simulink library "CommercialVehicleLibrary2G"  (R2021a)
settings: Solver=VariableStepAuto  StartTime=0.0  StopTime=10.0  RelTol=1e-3
values from neighbouring files (symbols this model uses):
  brake_input = [0   tmax ... (first row only)    [init_vehicle.m]    (also in run_Circle.m = [0  tmax; run_Coastdown.m = [0  2  tmax; run_DoubleLaneChangeDriver.m = [0   2  tmax; run_MaxAcc.m = [0  2  tmax)
  pose_t0 = [0 0 0 0]    [init_vehicle.m]    (also in run_Circle.m; run_Coastdown.m; run_DoubleLaneChangeDriver.m; run_MaxAcc.m)
  rdfname = 'TNO_FlatRoad.rdf'    [run_Circle.m]    (also in run_Coastdown.m; run_DoubleLaneChangeDriver.m; run_MaxAcc.m; run_Rollover.m)
  rdfname_inner = 'TNO_FlatRoad.rdf'    [run_Circle.m]    (also in run_Coastdown.m; run_DoubleLaneChangeDriver.m; run_MaxAcc.m; run_Rollover.m)
  steer_input = [0  tmax ... (first row only)    [init_vehicle.m]    (also in run_Circle.m = [0  2   10     13       tmax; run_Coastdown.m = [0 tmax; run_DoubleLaneChangeDriver.m = [0 tmax; run_MaxAcc.m = [0 tmax)
  throttle_input = [0         tmax ... (first row only)    [init_vehicle.m]    (also in run_Circle.m; run_Coastdown.m = [0        10         10.0001 tmax; run_DoubleLaneChangeDriver.m = [0        tmax; run_MaxAcc.m = [0        tmax)
  Vx = 0    [init_vehicle.m]    (also in run_Circle.m = Vx_kmh/3.6; run_Coastdown.m = Vx_kmh/3.6; run_DoubleLaneChangeDriver.m = Vx_kmh/3.6; run_MaxAcc.m)
  Vx_input = [0  tmax ... (first row only)    [init_vehicle.m]    (also in run_Circle.m; run_Coastdown.m = [0 tmax; run_DoubleLaneChangeDriver.m = [0 tmax; run_MaxAcc.m = [0 tmax)
undefined symbols (not defined in the file or in its folder): Drive, Floor, Fzstat, Fzstat1, Fzstat3, l, l_load1, l_load2, lbar, mass_load1, mass_load2, psi_semitrailer, rho, rim_Ixx, rim_Iyy, rim_mass, Steer, steer_path, tpfname, X, x_torsion, xcg, xcg1, xcg2, xcg_front, xcg_rear, xdrive1, xload1, xload2, xpos1, xref, xrev1, Xt0, Y, Yt0, Z
libraries: sm_lib x291, $bdroot x157, nesl_utility x143, vrlib x1
(part 8 of 12)

== system CommercialVehicleLibrary2G/Trailers/Trailer - 3 axle  ==
  Mb_trailer : Inport
  Bus Creator : BusCreator  Inputs=6
  Cameras : Subsystem  Commented=on
      settings: PortSchema="{\"entries\":[{\"content\":{\"sides\":[{\"content\":{\"connectorIds\":[]},\"type\":\"ConnectorPlacement.EquallySpacedRectSide\",\"uuid\":\"a276cb58-0a92-429b-8e88-be3307b37bb7\"},{\"content\":{\"connectorIds\":[],\"side\":\"RIGHT\"},\"type\":\"ConnectorPlacement.EquallySpacedRectSide\",\"uuid\":\"8a90bce0-2fe2-4c94-b803-8b8b0449a6a1\"},{\"content\":{\"connectorIds\":[],\"side\":\"TOP\"},\"type\":\"ConnectorPlacement.EquallySpacedRectSide\",\"uuid\":\"98d3107c-5bc7-4afe-b9f8-41acdc56c58c\"},{\"content\":{\"connectorIds\":[\"RConn1\"],\"side\":\"BOTTOM\"},\"type\":\"ConnectorPlacement.EquallySpacedRectSide\",\"uuid\":\"4e4e33e6-8433-45a0-a537-d9ee13bc0975\"}]},\"type\":\"ConnectorPlacement.EquallySpacedConnector\",\"uuid\":\"603d60ad-e553-44b7-87a5-94eb629e36a6\"}],\"packageUris\":[\"http://schema.mathworks.com/mf0/Connector/R2020b\"],\"version\":\"1.0\"}"
  Drawbar joint 1 : $bdroot/Components/Drawbar joint   SystemSampleTime=-1  VariantActivationTime=update diagram  Latency=0  AutoFrameSizeCalculation=off
  To origin : sm_lib/Frames and Transforms/Rigid Transform  TranslationMethod=Cartesian  TranslationStandardOffset=0  TranslationLengthUnit=m  TranslationStandardAxis=+Z  TranslationCartesianOffset=[-xcg2 0 -1.2]  TranslationROffset=0  TranslationROffsetUnits=m  TranslationZOffset=0  TranslationZOffsetUnits=m  TranslationThetaOffset=0  TranslationThetaOffsetUnits=deg  RotationMethod=None  RotationAngleUnits=deg  RotationStandardAxis=+Z  RotationAngle=0.0  RotationArbitraryAxis=[0 0 1]  FollAlignAxisA=+X  BaseAlignAxisA=+Y  FollAlignAxisB=+Y  BaseAlignAxisB=+Z  RotationSequenceAxes=FollowerAxes  RotationSequence=XYX  RotationSequenceAngles=[0 0 0]  RotationSequenceAnglesUnits=deg  RotationMatrix=[1 0 0; 0 1 0; 0 0 1]
  Trailer axle 1 : $bdroot/Assemblies/Trailer axle  xpos=0+xcg2  tpfname='truck3.tpf'  rdfname=rdfname  Vx=Vx  Fzstat=Fzstat
  Trailer axle 2 : $bdroot/Assemblies/Trailer axle  xpos=xpos2  tpfname='truck3.tpf'  rdfname=rdfname  Vx=Vx  Fzstat=Fzstat
  Trailer axle 3 : $bdroot/Assemblies/Trailer axle  xpos=xpos3  tpfname='truck3.tpf'  rdfname=rdfname  Vx=Vx  Fzstat=Fzstat
  Trailer load center : $bdroot/Assemblies/Trailer load center  xload=xcg1  zload=1.3  mass_load=0.5*mass_load  l_load=0.50*l_chassis  w=2.5  rho=rho
  Trailer load center1 : $bdroot/Assemblies/Trailer load center  xload=xcg2  zload=1.3  mass_load=0.5*mass_load  l_load=0.50*l_chassis  w=2.5  rho=rho
  Trailer_front : sm_lib/Body Elements/Brick Solid  GraphicAmbientColor=[0.15 0.15 0.15 1.0]  BasedOnType=Density  BrickDimensions=[l w h]  BrickDimensionUnits=m  CenterOfMass=[0 0 0]  CenterOfMassUnits=m  GraphicDiffuseColor=[0.9 0.9 0.9]  Density=1000  DensityUnits=kg/m^3  DoExposeReferenceFrame=on  GraphicEmissiveColor=[0.0 0.0 0.0 1.0]  ExportEntireGeometry=off  SerializedFrames=<Frames><Frame><Id>Frame1</Id><Value><Name>F1</Name><Origin><Source>ReferenceFrame</Source><FeatureName></FeatureName></Origin><PrimaryAxis><DefinedDirection>+Z</DefinedDirection><Source>ReferenceFrame</Source><SourceDirection>+Z</SourceDirection><FeatureName></FeatureName></PrimaryAxis><SecondaryAxis><DefinedDirection>+X</DefinedDirection><Source>ReferenceFrame</Source><SourceDirection>+X</SourceDirection><FeatureName></FeatureName></SecondaryAxis></Value></Frame></Frames>  MarkerShape=Sphere  MarkerSize=10  GraphicType=FromGeometry  InertiaType=Custom  Mass=chassis_mass  MassUnits=kg  MomentsOfInertia=[chassis_Ixx chassis_Iyy chassis_Izz]  MomentsOfInertiaUnits=kg*m^2  GraphicOpacity=0.8  ProductsOfInertia=[0 0 0]  ProductsOfInertiaUnits=kg*m^2  GraphicShininess=75  GraphicSpecularColor=[0.5 0.5 0.5 1.0]  GraphicVisPropType=SimpleVisualProperties
  Trailer_rear : sm_lib/Body Elements/Brick Solid  GraphicAmbientColor=[0.15 0.15 0.15 1.0]  BasedOnType=Density  BrickDimensions=[l w h]  BrickDimensionUnits=m  CenterOfMass=[0 0 0]  CenterOfMassUnits=m  GraphicDiffuseColor=[0.9 0.9 0.9]  Density=1000  DensityUnits=kg/m^3  DoExposeReferenceFrame=on  GraphicEmissiveColor=[0.0 0.0 0.0 1.0]  ExportEntireGeometry=off  SerializedFrames=<Frames><Frame><Id>Frame1</Id><Value><Name>F1</Name><Origin><Source>ReferenceFrame</Source><FeatureName></FeatureName></Origin><PrimaryAxis><DefinedDirection>+Z</DefinedDirection><Source>ReferenceFrame</Source><SourceDirection>+Z</SourceDirection><FeatureName></FeatureName></PrimaryAxis><SecondaryAxis><DefinedDirection>+X</DefinedDirection><Source>ReferenceFrame</Source><SourceDirection>+X</SourceDirection><FeatureName></FeatureName></SecondaryAxis></Value></Frame></Frames>  MarkerShape=Sphere  MarkerSize=10  GraphicType=FromGeometry  InertiaType=Custom  Mass=chassis_mass  MassUnits=kg  MomentsOfInertia=[chassis_Ixx chassis_Iyy chassis_Izz]  MomentsOfInertiaUnits=kg*m^2  GraphicOpacity=0.8  ProductsOfInertia=[0 0 0]  ProductsOfInertiaUnits=kg*m^2  GraphicShininess=75  GraphicSpecularColor=[0.5 0.5 0.5 1.0]  GraphicVisPropType=SimpleVisualProperties
  Trailer_torsion : $bdroot/Components/Trailer_torsion  SystemSampleTime=-1  VariantActivationTime=update diagram  Latency=0  AutoFrameSizeCalculation=off
      settings: PortSchema="{\"entries\":[{\"content\":{\"sides\":[{\"content\":{\"connectorIds\":[\"LConn1\"]},\"type\":\"ConnectorPlacement.EquallySpacedRectSide\",\"uuid\":\"b43c74bd-af15-4ffb-863b-6a132848d787\"},{\"content\":{\"connectorIds\":[\"RConn1\"],\"side\":\"RIGHT\"},\"type\":\"ConnectorPlacement.EquallySpacedRectSide\",\"uuid\":\"8ef5ae9f-2f99-4b38-816f-c2fb0756fe1b\"},{\"content\":{\"connectorIds\":[\"Out1\"],\"side\":\"TOP\"},\"type\":\"ConnectorPlacement.EquallySpacedRectSide\",\"uuid\":\"649c363b-e78d-45fa-ac8c-bda3eda724e3\"}]},\"type\":\"ConnectorPlacement.EquallySpacedConnector\",\"uuid\":\"06fb9ebd-5177-4420-93bb-82569f181fb4\"}],\"packageUris\":[\"http://schema.mathworks.com/mf0/Connector/R2020b\"],\"version\":\"1.0\"}"
  Pin Coupling : PMIOPort  Tag=PMCPort  Side=Left
  Connection : PMIOPort  Tag=PMCPort  Port=2  Side=Right
  Signals : Outport
  wires:
  [axle2] -> Bus Creator/2  "axle2"
  [axle1] -> Bus Creator/1  "axle1"
  Bus Creator/1 -> Signals/1
  Trailer load center1/1 -> [semitrailerload2]
  Trailer_torsion/1 -> [torsion]
  Mb_trailer/1 -> Trailer axle 1/1, Trailer axle 2/1, Trailer axle 3/1
  Trailer axle 2/1 -> [axle2]
  Trailer load center/1 -> [semitrailerload1]
  Trailer axle 1/1 -> [axle1]
  Trailer axle 3/1 -> [axle3]
  [semitrailerload1] -> Bus Creator/4  "load1"
  [semitrailerload2] -> Bus Creator/5  "load2"
  [torsion] -> Bus Creator/6  "torsion"
  [axle3] -> Bus Creator/3  "axle3"
  connections:
  To origin/LConn1 -- Trailer load center1/LConn1 -- Trailer axle 2/LConn1 -- Trailer axle 3/LConn1 -- Trailer_rear/LConn1
  Cameras/RConn1 -- Trailer_front/LConn1 -- Trailer_torsion/LConn1 -- Trailer load center/LConn1
  Trailer_rear/RConn1 -- Trailer_torsion/RConn1
  To origin/RConn1 -- Connection/RConn1
  Pin Coupling/RConn1 -- Drawbar joint 1/LConn1
  Drawbar joint 1/RConn1 -- Trailer_front/RConn1
  Drawbar joint 1/RConn2 -- Trailer axle 1/LConn1

== system CommercialVehicleLibrary2G/Utilities/Differentiator//filter ==
  pos : Inport
  Gain : Gain  Gain=c  SaturateOnIntegerOverflow=on  OutDataTypeStr=Inherit: Same as input  ParamDataTypeStr=Inherit: Same as input
  Gain2 : Gain  Gain=2*sqrt(c)  SaturateOnIntegerOverflow=on  OutDataTypeStr=Inherit: Same as input  ParamDataTypeStr=Inherit: Same as input
  Integrator2 : Integrator
  Integrator3 : Integrator
  Sum1 : Sum  Inputs=-+|  SaturateOnIntegerOverflow=on
  Sum2 : Sum  Inputs=-+|  SaturateOnIntegerOverflow=on
  actual pos : Outport
  wires:
  Integrator2/1 -> Integrator3/1, Gain2/1
  Integrator3/1 -> Sum2/1, actual pos/1
  Sum1/1 -> Integrator2/1
  Sum2/1 -> Gain/1
  pos/1 -> Sum2/2
  Gain2/1 -> Sum1/1
  Gain/1 -> Sum1/2

== system CommercialVehicleLibrary2G/Utilities/Non-moving road ==
  omega2 : Constant  Value=zeros(18,1)
  road : Outport
  wires:
  omega2/1 -> road/1

== system CommercialVehicleLibrary2G/Utilities/Scaling factors ==
  s_LKX : Constant  Value=LKX
  s_LKY : Constant  Value=LKY
  s_LKYC : Constant  Value=LKYC
  s_LKZC : Constant  Value=LKZC
  s_LMUX : Constant  Value=LMUX
  s_LMUY : Constant  Value=LMUY
  s_LTR : Constant  Value=LTR
  scaling_vector : Mux  Inputs=7
  scaling : Outport
  wires:
  s_LMUX/1 -> scaling_vector/1
  s_LKX/1 -> scaling_vector/2
  s_LMUY/1 -> scaling_vector/3
  s_LKY/1 -> scaling_vector/4
  s_LKYC/1 -> scaling_vector/5
  s_LTR/1 -> scaling_vector/6
  s_LKZC/1 -> scaling_vector/7
  scaling_vector/1 -> scaling/1

== system CommercialVehicleLibrary2G/Utilities/To_workspace_dolly ==
  note: Axle 1
  note: Axle 2
  note: Tyres & Omega
  In1 : Inport
  Bus Selector10 : BusSelector  OutputSignals=axle1.Axle_roll  OutputAsBus=on
  Bus Selector12 : BusSelector  OutputSignals=axle2.Axle_acc  OutputAsBus=on
  Bus Selector2 : BusSelector  OutputSignals=axle2.Axle_pos  OutputAsBus=on
  Bus Selector3 : BusSelector  OutputSignals=axle2.Axle_roll  OutputAsBus=on
  Bus Selector5 : BusSelector  OutputSignals=axle1.Axle_pos  OutputAsBus=on
  Bus Selector6 : BusSelector  OutputSignals=axle1.Axle_acc  OutputAsBus=on
  Subsystem : Subsystem
  Subsystem1 : Subsystem
  Subsystem2 : Subsystem
  Subsystem3 : Subsystem
  To Workspace10 : ToWorkspace  VariableName=p_trailer1_axle2_acc  SampleTime=-1
  To Workspace23 : ToWorkspace  VariableName=p_trailer1_axle1_roll  SampleTime=-1
  To Workspace30 : ToWorkspace  VariableName=p_trailer1_Fx  SampleTime=-1
  To Workspace31 : ToWorkspace  VariableName=p_trailer1_Fy  SampleTime=-1
  To Workspace4 : ToWorkspace  VariableName=p_trailer1_axle2_roll  SampleTime=-1
  To Workspace5 : ToWorkspace  VariableName=p_trailer1_axle1_pos  SampleTime=-1
  To Workspace6 : ToWorkspace  VariableName=p_trailer1_axle1_acc  SampleTime=-1
  To Workspace7 : ToWorkspace  VariableName=p_trailer1_omega  SampleTime=-1
  To Workspace8 : ToWorkspace  VariableName=p_trailer1_axle2_pos  SampleTime=-1
  To Workspace9 : ToWorkspace  VariableName=p_trailer1_Fz  SampleTime=-1
  wires:
  Bus Selector10/1 -> To Workspace23/1
  In1/1 -> Bus Selector3/1, Bus Selector2/1, Bus Selector5/1, Bus Selector12/1, Bus Selector10/1, Subsystem3/1(In1), Subsystem2/1(In1), Subsystem1/1(In1), Subsystem/1(In1), Bus Selector6/1
  Bus Selector12/1 -> To Workspace10/1
  Bus Selector6/1 -> To Workspace6/1
  Bus Selector5/1 -> To Workspace5/1
  Subsystem3/1(Out1) -> To Workspace7/1
  Subsystem2/1(Out1) -> To Workspace9/1
  Subsystem1/1(Out1) -> To Workspace31/1
  Subsystem/1(Out1) -> To Workspace30/1
  Bus Selector3/1 -> To Workspace4/1
  Bus Selector2/1 -> To Workspace8/1

== system CommercialVehicleLibrary2G/Utilities/To_workspace_drawbar_trailer_2axle ==
  note: Axle 1
  note: Axle 2
  note: Chassis & Load
  note: Tyres & Omega
  In1 : Inport
  Bus Selector10 : BusSelector  OutputSignals=axle1.Axle_roll  OutputAsBus=on
  Bus Selector11 : BusSelector  OutputSignals=trailerload.acc_center  OutputAsBus=on
  Bus Selector12 : BusSelector  OutputSignals=axle2.Axle_acc  OutputAsBus=on
  Bus Selector2 : BusSelector  OutputSignals=axle2.Axle_pos  OutputAsBus=on
  Bus Selector22 : BusSelector  OutputSignals=trailerload.pos  OutputAsBus=on
  Bus Selector3 : BusSelector  OutputSignals=axle2.Axle_roll  OutputAsBus=on
  Bus Selector5 : BusSelector  OutputSignals=axle1.Axle_pos  OutputAsBus=on
  Bus Selector6 : BusSelector  OutputSignals=axle1.Axle_acc  OutputAsBus=on
  Bus Selector7 : BusSelector  OutputSignals=trailerload.acc_corner  OutputAsBus=on
  Subsystem : Subsystem
  Subsystem1 : Subsystem
  Subsystem2 : Subsystem
  Subsystem3 : Subsystem
  To Workspace1 : ToWorkspace  VariableName=p_trailer1_load_pos  SampleTime=-1
  To Workspace10 : ToWorkspace  VariableName=p_trailer1_axle2_acc  SampleTime=-1
  To Workspace2 : ToWorkspace  VariableName=p_trailer1_load_acc_center  SampleTime=-1
  To Workspace23 : ToWorkspace  VariableName=p_trailer1_axle1_roll  SampleTime=-1
  To Workspace3 : ToWorkspace  VariableName=p_trailer1_load_acc_corner  SampleTime=-1
  To Workspace30 : ToWorkspace  VariableName=p_trailer1_Fx  SampleTime=-1
  To Workspace31 : ToWorkspace  VariableName=p_trailer1_Fy  SampleTime=-1
  To Workspace4 : ToWorkspace  VariableName=p_trailer1_axle2_roll  SampleTime=-1
  To Workspace5 : ToWorkspace  VariableName=p_trailer1_axle1_pos  SampleTime=-1
  To Workspace6 : ToWorkspace  VariableName=p_trailer1_axle1_acc  SampleTime=-1
  To Workspace7 : ToWorkspace  VariableName=p_trailer1_omega  SampleTime=-1
  To Workspace8 : ToWorkspace  VariableName=p_trailer1_axle2_pos  SampleTime=-1
  To Workspace9 : ToWorkspace  VariableName=p_trailer1_Fz  SampleTime=-1
  wires:
  Bus Selector7/1 -> To Workspace3/1
  Bus Selector10/1 -> To Workspace23/1
  Bus Selector22/1 -> To Workspace1/1
  In1/1 -> Bus Selector3/1, Bus Selector2/1, Bus Selector5/1, Bus Selector12/1, Bus Selector10/1, Subsystem3/1(In1), Bus Selector7/1, Subsystem2/1(In1), Subsystem1/1(In1), Bus Selector22/1, Subsystem/1(In1), Bus Selector11/1, Bus Selector6/1
  Bus Selector12/1 -> To Workspace10/1
  Bus Selector6/1 -> To Workspace6/1
  Bus Selector5/1 -> To Workspace5/1
  Subsystem3/1(Out1) -> To Workspace7/1
  Subsystem2/1(Out1) -> To Workspace9/1
  Subsystem1/1(Out1) -> To Workspace31/1
  Subsystem/1(Out1) -> To Workspace30/1
  Bus Selector3/1 -> To Workspace4/1
  Bus Selector2/1 -> To Workspace8/1
  Bus Selector11/1 -> To Workspace2/1

== system CommercialVehicleLibrary2G/Utilities/To_workspace_drawbar_trailer_3axle ==
  note: Axle 1
  note: Axle 2
  note: Chassis & Load
  note: Tyres & Omega
  note: Axle 3
  In1 : Inport
  Bus Selector1 : BusSelector  OutputSignals=axle3.Axle_roll  OutputAsBus=on
  Bus Selector10 : BusSelector  OutputSignals=axle1.Axle_roll  OutputAsBus=on
  Bus Selector11 : BusSelector  OutputSignals=trailerload.acc_center  OutputAsBus=on
  Bus Selector12 : BusSelector  OutputSignals=axle2.Axle_acc  OutputAsBus=on
  Bus Selector2 : BusSelector  OutputSignals=axle2.Axle_pos  OutputAsBus=on
  Bus Selector22 : BusSelector  OutputSignals=trailerload.pos  OutputAsBus=on
  Bus Selector3 : BusSelector  OutputSignals=axle2.Axle_roll  OutputAsBus=on
  Bus Selector4 : BusSelector  OutputSignals=axle3.Axle_pos  OutputAsBus=on
  Bus Selector5 : BusSelector  OutputSignals=axle1.Axle_pos  OutputAsBus=on
  Bus Selector6 : BusSelector  OutputSignals=axle1.Axle_acc  OutputAsBus=on
  Bus Selector7 : BusSelector  OutputSignals=trailerload.acc_corner  OutputAsBus=on
  Bus Selector8 : BusSelector  OutputSignals=axle3.Axle_acc  OutputAsBus=on
  Subsystem : Subsystem
  Subsystem1 : Subsystem
  Subsystem2 : Subsystem
  Subsystem3 : Subsystem
  To Workspace1 : ToWorkspace  VariableName=p_trailer1_load_pos  SampleTime=-1
  To Workspace10 : ToWorkspace  VariableName=p_trailer1_axle2_acc  SampleTime=-1
  To Workspace11 : ToWorkspace  VariableName=p_trailer1_axle3_pos  SampleTime=-1
  To Workspace12 : ToWorkspace  VariableName=p_trailer1_axle3_acc  SampleTime=-1
  To Workspace13 : ToWorkspace  VariableName=p_trailer1_load_acc_corner  SampleTime=-1
  To Workspace2 : ToWorkspace  VariableName=p_trailer1_load_acc_center  SampleTime=-1
  To Workspace23 : ToWorkspace  VariableName=p_trailer1_axle1_roll  SampleTime=-1
  To Workspace3 : ToWorkspace  VariableName=p_trailer1_axle3_roll  SampleTime=-1
  To Workspace30 : ToWorkspace  VariableName=p_trailer1_Fx  SampleTime=-1
  To Workspace31 : ToWorkspace  VariableName=p_trailer1_Fy  SampleTime=-1
  To Workspace4 : ToWorkspace  VariableName=p_trailer1_axle2_roll  SampleTime=-1
  To Workspace5 : ToWorkspace  VariableName=p_trailer1_axle1_pos  SampleTime=-1
  To Workspace6 : ToWorkspace  VariableName=p_trailer1_axle1_acc  SampleTime=-1
  To Workspace7 : ToWorkspace  VariableName=p_trailer1_omega  SampleTime=-1
  To Workspace8 : ToWorkspace  VariableName=p_trailer1_axle2_pos  SampleTime=-1
  To Workspace9 : ToWorkspace  VariableName=p_trailer1_Fz  SampleTime=-1
  wires:
  Bus Selector7/1 -> To Workspace13/1
  Bus Selector10/1 -> To Workspace23/1
  Bus Selector22/1 -> To Workspace1/1
  In1/1 -> Bus Selector3/1, Bus Selector2/1, Bus Selector5/1, Bus Selector12/1, Bus Selector10/1, Bus Selector8/1, Bus Selector4/1, Bus Selector1/1, Subsystem3/1(In1), Bus Selector7/1, Subsystem2/1(In1), Subsystem1/1(In1), Bus Selector22/1, Subsystem/1(In1), Bus Selector11/1, Bus Selector6/1
  Bus Selector12/1 -> To Workspace10/1
  Bus Selector6/1 -> To Workspace6/1
  Bus Selector5/1 -> To Workspace5/1
  Subsystem3/1(Out1) -> To Workspace7/1
  Subsystem2/1(Out1) -> To Workspace9/1
  Subsystem1/1(Out1) -> To Workspace31/1
  Subsystem/1(Out1) -> To Workspace30/1
  Bus Selector3/1 -> To Workspace4/1
  Bus Selector2/1 -> To Workspace8/1
  Bus Selector11/1 -> To Workspace2/1
  Bus Selector4/1 -> To Workspace11/1
  Bus Selector8/1 -> To Workspace12/1
  Bus Selector1/1 -> To Workspace3/1

== system CommercialVehicleLibrary2G/Utilities/To_workspace_semitrailer ==
  note: Axle 1
  note: Axle 2
  note: Axle 3
  note: Tyres & Omega
  In1 : Inport
  Bus Selector1 : BusSelector  OutputSignals=axle1.Axle_roll  OutputAsBus=on
  Bus Selector11 : BusSelector  OutputSignals=axle3.Axle_acc  OutputAsBus=on
  Bus Selector2 : BusSelector  OutputSignals=axle2.Axle_pos  OutputAsBus=on
  Bus Selector22 : BusSelector  OutputSignals=axle3.Axle_pos  OutputAsBus=on
  Bus Selector3 : BusSelector  OutputSignals=axle2.Axle_acc  OutputAsBus=on
  Bus Selector4 : BusSelector  OutputSignals=axle2.Axle_roll  OutputAsBus=on
  Bus Selector5 : BusSelector  OutputSignals=axle1.Axle_pos  OutputAsBus=on
  Bus Selector6 : BusSelector  OutputSignals=axle1.Axle_acc  OutputAsBus=on
  Bus Selector7 : BusSelector  OutputSignals=axle3.Axle_roll  OutputAsBus=on
  Subsystem : Subsystem
  Subsystem1 : Subsystem
  Subsystem2 : Subsystem
  Subsystem3 : Subsystem
  To Workspace1 : ToWorkspace  VariableName=p_semitraileraxle3_pos  SampleTime=-1
  To Workspace10 : ToWorkspace  VariableName=p_semitraileraxle2_pos  SampleTime=-1
  To Workspace11 : ToWorkspace  VariableName=p_semitraileraxle2_acc  SampleTime=-1
  To Workspace2 : ToWorkspace  VariableName=p_semitraileraxle3_acc  SampleTime=-1
  To Workspace3 : ToWorkspace  VariableName=p_semitraileraxle3_roll  SampleTime=-1
  To Workspace30 : ToWorkspace  VariableName=p_semitrailer_Fx  SampleTime=-1
  To Workspace31 : ToWorkspace  VariableName=p_semitrailer_Fy  SampleTime=-1
  To Workspace4 : ToWorkspace  VariableName=p_semitraileraxle1_roll  SampleTime=-1
  To Workspace5 : ToWorkspace  VariableName=p_semitraileraxle1_pos  SampleTime=-1
  To Workspace6 : ToWorkspace  VariableName=p_semitraileraxle1_acc  SampleTime=-1
  To Workspace7 : ToWorkspace  VariableName=p_semitrailer_omega  SampleTime=-1
  To Workspace8 : ToWorkspace  VariableName=p_semitraileraxle2_roll  SampleTime=-1
  To Workspace9 : ToWorkspace  VariableName=p_semitrailer_Fz  SampleTime=-1
  wires:
  Bus Selector22/1 -> To Workspace1/1
  Bus Selector6/1 -> To Workspace6/1
  Bus Selector5/1 -> To Workspace5/1
  Subsystem3/1(Out1) -> To Workspace7/1
  Subsystem2/1(Out1) -> To Workspace9/1
  Subsystem1/1(Out1) -> To Workspace31/1
  Subsystem/1(Out1) -> To Workspace30/1
  Bus Selector3/1 -> To Workspace11/1
  Bus Selector2/1 -> To Workspace10/1
  Bus Selector11/1 -> To Workspace2/1
  Bus Selector1/1 -> To Workspace4/1
  Bus Selector4/1 -> To Workspace8/1
  In1/1 -> Bus Selector3/1, Bus Selector2/1, Bus Selector5/1, Bus Selector7/1, Subsystem3/1(In1), Subsystem2/1(In1), Subsystem1/1(In1), Bus Selector22/1, Subsystem/1(In1), Bus Selector11/1, Bus Selector4/1, Bus Selector1/1, Bus Selector6/1
  Bus Selector7/1 -> To Workspace3/1

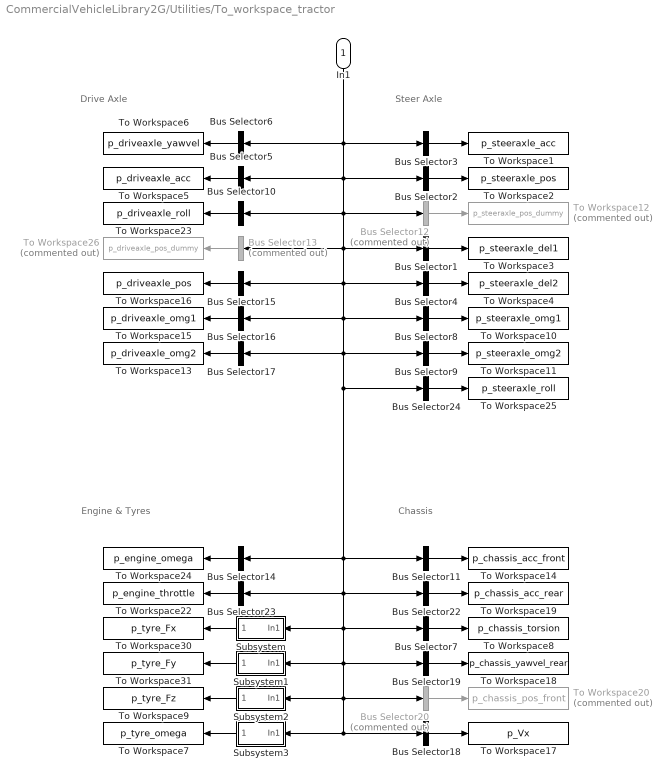
== system CommercialVehicleLibrary2G/Utilities/To_workspace_tractor ==
  note: Drive Axle
  note: Steer Axle
  note: Chassis
  note: Engine & Tyres
  In1 : Inport
  Bus Selector1 : BusSelector  OutputSignals=steeraxle.Delta 1_L  OutputAsBus=on
  Bus Selector10 : BusSelector  OutputSignals=driveaxle.roll  OutputAsBus=on
  Bus Selector11 : BusSelector  OutputSignals=chassis.front_acc  OutputAsBus=on
  Bus Selector12 : BusSelector  Commented=on  OutputSignals=steeraxle.Dummyaxle_pos  OutputAsBus=on
  Bus Selector13 : BusSelector  Commented=on  OutputSignals=driveaxle.G2_Driveaxle_pos_dummy  OutputAsBus=on
  Bus Selector14 : BusSelector  OutputSignals=driveline.omega  OutputAsBus=on
  Bus Selector15 : BusSelector  OutputSignals=driveaxle.pos  OutputAsBus=on
  Bus Selector16 : BusSelector  OutputSignals=driveaxle.Omega1  OutputAsBus=on
  Bus Selector17 : BusSelector  OutputSignals=driveaxle.Omega2  OutputAsBus=on
  Bus Selector18 : BusSelector  OutputSignals=chassis.Vx  OutputAsBus=on
  Bus Selector19 : BusSelector  OutputSignals=chassis.yawvel  OutputAsBus=on
  Bus Selector2 : BusSelector  OutputSignals=steeraxle.pos  OutputAsBus=on
  Bus Selector20 : BusSelector  Commented=on  OutputSignals=chassis.pos_chassis frt  OutputAsBus=on
  Bus Selector22 : BusSelector  OutputSignals=chassis.centre_acc  OutputAsBus=on
  Bus Selector23 : BusSelector  OutputSignals=driveline.throttle  OutputAsBus=on
  Bus Selector24 : BusSelector  OutputSignals=steeraxle.roll  OutputAsBus=on
  Bus Selector3 : BusSelector  OutputSignals=steeraxle.acc  OutputAsBus=on
  Bus Selector4 : BusSelector  OutputSignals=steeraxle.Delta 2_R  OutputAsBus=on
  Bus Selector5 : BusSelector  OutputSignals=driveaxle.acc  OutputAsBus=on
  Bus Selector6 : BusSelector  OutputSignals=chassis.yawvel  OutputAsBus=on
  Bus Selector7 : BusSelector  OutputSignals=chassis.torsion  OutputAsBus=on
  Bus Selector8 : BusSelector  OutputSignals=steeraxle.Omega1  OutputAsBus=on
  Bus Selector9 : BusSelector  OutputSignals=steeraxle.Omega2  OutputAsBus=on
  Subsystem : Subsystem
  Subsystem1 : Subsystem
  Subsystem2 : Subsystem
  Subsystem3 : Subsystem
  To Workspace1 : ToWorkspace  VariableName=p_steeraxle_acc  SampleTime=-1
  To Workspace10 : ToWorkspace  VariableName=p_steeraxle_omg1  SampleTime=-1
  To Workspace11 : ToWorkspace  VariableName=p_steeraxle_omg2  SampleTime=-1
  To Workspace12 : ToWorkspace  Commented=on  VariableName=p_steeraxle_pos_dummy  SampleTime=-1
  To Workspace13 : ToWorkspace  VariableName=p_driveaxle_omg2  SampleTime=-1
  To Workspace14 : ToWorkspace  VariableName=p_chassis_acc_front  SampleTime=-1
  To Workspace15 : ToWorkspace  VariableName=p_driveaxle_omg1  SampleTime=-1
  To Workspace16 : ToWorkspace  VariableName=p_driveaxle_pos  SampleTime=-1
  To Workspace17 : ToWorkspace  VariableName=p_Vx  SampleTime=-1
  To Workspace18 : ToWorkspace  VariableName=p_chassis_yawvel_rear  SampleTime=-1
  To Workspace19 : ToWorkspace  VariableName=p_chassis_acc_rear  SampleTime=-1
  To Workspace2 : ToWorkspace  VariableName=p_steeraxle_pos  SampleTime=-1
  To Workspace20 : ToWorkspace  Commented=on  VariableName=p_chassis_pos_front  SampleTime=-1
  To Workspace22 : ToWorkspace  VariableName=p_engine_throttle  SampleTime=-1
  To Workspace23 : ToWorkspace  VariableName=p_driveaxle_roll  SampleTime=-1
  To Workspace24 : ToWorkspace  VariableName=p_engine_omega  SampleTime=-1
  To Workspace25 : ToWorkspace  VariableName=p_steeraxle_roll  SampleTime=-1
  To Workspace26 : ToWorkspace  Commented=on  VariableName=p_driveaxle_pos_dummy  SampleTime=-1
  To Workspace3 : ToWorkspace  VariableName=p_steeraxle_del1  SampleTime=-1
  To Workspace30 : ToWorkspace  VariableName=p_tyre_Fx  SampleTime=-1
  To Workspace31 : ToWorkspace  VariableName=p_tyre_Fy  SampleTime=-1
  To Workspace4 : ToWorkspace  VariableName=p_steeraxle_del2  SampleTime=-1
  To Workspace5 : ToWorkspace  VariableName=p_driveaxle_acc  SampleTime=-1
  To Workspace6 : ToWorkspace  VariableName=p_driveaxle_yawvel  SampleTime=-1
  To Workspace7 : ToWorkspace  VariableName=p_tyre_omega  SampleTime=-1
  To Workspace8 : ToWorkspace  VariableName=p_chassis_torsion  SampleTime=-1
  To Workspace9 : ToWorkspace  VariableName=p_tyre_Fz  SampleTime=-1
  wires:
  Bus Selector13/1 -> To Workspace26/1
  Bus Selector24/1 -> To Workspace25/1
  Bus Selector10/1 -> To Workspace23/1
  Bus Selector23/1 -> To Workspace22/1
  Bus Selector20/1 -> To Workspace20/1
  In1/1 -> Bus Selector3/1, Bus Selector2/1, Bus Selector5/1, Bus Selector12/1, Bus Selector10/1, Bus Selector1/1, Bus Selector13/1, Bus Selector4/1, Bus Selector15/1, Bus Selector8/1, Bus Selector16/1, Bus Selector9/1, Bus Selector17/1, Bus Selector11/1, Bus Selector14/1, Bus Selector22/1, Bus Selector7/1, Subsystem/1(In1), Bus Selector19/1, Subsystem1/1(In1), Bus Selector20/1, Subsystem2/1(In1), Subsystem3/1(In1), Bus Selector18/1, Bus Selector23/1, Bus Selector24/1, Bus Selector6/1
  Bus Selector22/1 -> To Workspace19/1
  Bus Selector19/1 -> To Workspace18/1
  Bus Selector15/1 -> To Workspace16/1
  Bus Selector17/1 -> To Workspace13/1
  Bus Selector16/1 -> To Workspace15/1
  Bus Selector12/1 -> To Workspace12/1
  Bus Selector9/1 -> To Workspace11/1
  Bus Selector8/1 -> To Workspace10/1
  Bus Selector6/1 -> To Workspace6/1
  Bus Selector5/1 -> To Workspace5/1
  Bus Selector4/1 -> To Workspace4/1
  Bus Selector1/1 -> To Workspace3/1
  Subsystem3/1(Out1) -> To Workspace7/1
  Subsystem2/1(Out1) -> To Workspace9/1
  Subsystem1/1(Out1) -> To Workspace31/1
  Subsystem/1(Out1) -> To Workspace30/1
  Bus Selector3/1 -> To Workspace1/1
  Bus Selector2/1 -> To Workspace2/1
  Bus Selector7/1 -> To Workspace8/1
  Bus Selector18/1 -> To Workspace17/1
  Bus Selector11/1 -> To Workspace14/1
  Bus Selector14/1 -> To Workspace24/1

== system CommercialVehicleLibrary2G/Utilities/To_workspace_trailer_2axle ==
  note: Axle 1
  note: Axle 2
  note: Chassis & Load
  note: Tyres & Omega
  In1 : Inport
  Bus Selector1 : BusSelector  OutputSignals=load2.acc_center  OutputAsBus=on
  Bus Selector10 : BusSelector  OutputSignals=axle1.Axle_roll  OutputAsBus=on
  Bus Selector11 : BusSelector  OutputSignals=load1.acc_center  OutputAsBus=on
  Bus Selector12 : BusSelector  OutputSignals=axle2.Axle_acc  OutputAsBus=on
  Bus Selector2 : BusSelector  OutputSignals=axle2.Axle_pos  OutputAsBus=on
  Bus Selector22 : BusSelector  OutputSignals=load1.pos  OutputAsBus=on
  Bus Selector3 : BusSelector  OutputSignals=axle2.Axle_roll  OutputAsBus=on
  Bus Selector4 : BusSelector  OutputSignals=load2.pos  OutputAsBus=on
  Bus Selector5 : BusSelector  OutputSignals=axle1.Axle_pos  OutputAsBus=on
  Bus Selector6 : BusSelector  OutputSignals=axle1.Axle_acc  OutputAsBus=on
  Bus Selector7 : BusSelector  OutputSignals=torsion  OutputAsBus=on
  Bus Selector8 : BusSelector  OutputSignals=load1.acc_corner  OutputAsBus=on
  Bus Selector9 : BusSelector  OutputSignals=load2.acc_corner  OutputAsBus=on
  Subsystem : Subsystem
  Subsystem1 : Subsystem
  Subsystem2 : Subsystem
  Subsystem3 : Subsystem
  To Workspace1 : ToWorkspace  VariableName=p_trailer1_load1_pos  SampleTime=-1
  To Workspace10 : ToWorkspace  VariableName=p_trailer1_axle2_acc  SampleTime=-1
  To Workspace11 : ToWorkspace  VariableName=p_trailer1_load2_pos  SampleTime=-1
  To Workspace12 : ToWorkspace  VariableName=p_trailer1_load2_acc_center  SampleTime=-1
  To Workspace13 : ToWorkspace  VariableName=p_trailer1_load1_acc_corner  SampleTime=-1
  To Workspace14 : ToWorkspace  VariableName=p_trailer1_load2_acc_corner  SampleTime=-1
  To Workspace2 : ToWorkspace  VariableName=p_trailer1_load1_acc_center  SampleTime=-1
  To Workspace23 : ToWorkspace  VariableName=p_trailer1_axle1_roll  SampleTime=-1
  To Workspace3 : ToWorkspace  VariableName=p_trailer1_torsion  SampleTime=-1
  To Workspace30 : ToWorkspace  VariableName=p_trailer1_Fx  SampleTime=-1
  To Workspace31 : ToWorkspace  VariableName=p_trailer1_Fy  SampleTime=-1
  To Workspace4 : ToWorkspace  VariableName=p_trailer1_axle2_roll  SampleTime=-1
  To Workspace5 : ToWorkspace  VariableName=p_trailer1_axle1_pos  SampleTime=-1
  To Workspace6 : ToWorkspace  VariableName=p_trailer1_axle1_acc  SampleTime=-1
  To Workspace7 : ToWorkspace  VariableName=p_trailer1_omega  SampleTime=-1
  To Workspace8 : ToWorkspace  VariableName=p_trailer1_axle2_pos  SampleTime=-1
  To Workspace9 : ToWorkspace  VariableName=p_trailer1_Fz  SampleTime=-1
  wires:
  Bus Selector9/1 -> To Workspace14/1
  Bus Selector8/1 -> To Workspace13/1
  Bus Selector10/1 -> To Workspace23/1
  Bus Selector22/1 -> To Workspace1/1
  Bus Selector12/1 -> To Workspace10/1
  Bus Selector6/1 -> To Workspace6/1
  Bus Selector5/1 -> To Workspace5/1
  Subsystem3/1(Out1) -> To Workspace7/1
  Subsystem2/1(Out1) -> To Workspace9/1
  Subsystem1/1(Out1) -> To Workspace31/1
  Subsystem/1(Out1) -> To Workspace30/1
  Bus Selector3/1 -> To Workspace4/1
  Bus Selector2/1 -> To Workspace8/1
  Bus Selector11/1 -> To Workspace2/1
  Bus Selector7/1 -> To Workspace3/1
  Bus Selector1/1 -> To Workspace12/1
  In1/1 -> Bus Selector3/1, Bus Selector2/1, Bus Selector5/1, Bus Selector12/1, Bus Selector10/1, Subsystem1/1(In1), Subsystem2/1(In1), Subsystem3/1(In1), Bus Selector4/1, Bus Selector7/1, Bus Selector9/1, Bus Selector1/1, Bus Selector22/1, Bus Selector8/1, Subsystem/1(In1), Bus Selector11/1, Bus Selector6/1
  Bus Selector4/1 -> To Workspace11/1

== system CommercialVehicleLibrary2G/Utilities/To_workspace_trailer_3axle ==
  note: Axle 1
  note: Axle 2
  note: Chassis & Load
  note: Tyres & Omega
  note: Axle 3
  In1 : Inport
  Bus Selector1 : BusSelector  OutputSignals=load2.acc_center  OutputAsBus=on
  Bus Selector10 : BusSelector  OutputSignals=axle1.Axle_roll  OutputAsBus=on
  Bus Selector11 : BusSelector  OutputSignals=load1.acc_center  OutputAsBus=on
  Bus Selector12 : BusSelector  OutputSignals=axle2.Axle_acc  OutputAsBus=on
  Bus Selector13 : BusSelector  OutputSignals=axle3.Axle_acc  OutputAsBus=on
  Bus Selector14 : BusSelector  OutputSignals=load1.acc_corner  OutputAsBus=on
  Bus Selector15 : BusSelector  OutputSignals=load2.acc_corner  OutputAsBus=on
  Bus Selector2 : BusSelector  OutputSignals=axle2.Axle_pos  OutputAsBus=on
  Bus Selector22 : BusSelector  OutputSignals=load1.pos  OutputAsBus=on
  Bus Selector3 : BusSelector  OutputSignals=axle2.Axle_roll  OutputAsBus=on
  Bus Selector4 : BusSelector  OutputSignals=load2.pos  OutputAsBus=on
  Bus Selector5 : BusSelector  OutputSignals=axle1.Axle_pos  OutputAsBus=on
  Bus Selector6 : BusSelector  OutputSignals=axle1.Axle_acc  OutputAsBus=on
  Bus Selector7 : BusSelector  OutputSignals=torsion  OutputAsBus=on
  Bus Selector8 : BusSelector  OutputSignals=axle3.Axle_roll  OutputAsBus=on
  Bus Selector9 : BusSelector  OutputSignals=axle3.Axle_pos  OutputAsBus=on
  Subsystem : Subsystem
  Subsystem1 : Subsystem
  Subsystem2 : Subsystem
  Subsystem3 : Subsystem
  To Workspace1 : ToWorkspace  VariableName=p_trailer1_load1_pos  SampleTime=-1
  To Workspace10 : ToWorkspace  VariableName=p_trailer1_axle2_acc  SampleTime=-1
  To Workspace11 : ToWorkspace  VariableName=p_trailer1_load2_pos  SampleTime=-1
  To Workspace12 : ToWorkspace  VariableName=p_trailer1_load2_acc_center  SampleTime=-1
  To Workspace13 : ToWorkspace  VariableName=p_trailer1_axle3_roll  SampleTime=-1
  To Workspace14 : ToWorkspace  VariableName=p_trailer1_axle3_pos  SampleTime=-1
  To Workspace15 : ToWorkspace  VariableName=p_trailer1_axle3_acc  SampleTime=-1
  To Workspace16 : ToWorkspace  VariableName=p_trailer1_load1_acc_corner  SampleTime=-1
  To Workspace17 : ToWorkspace  VariableName=p_trailer1_load2_acc_corner  SampleTime=-1
  To Workspace2 : ToWorkspace  VariableName=p_trailer1_load1_acc_center  SampleTime=-1
  To Workspace23 : ToWorkspace  VariableName=p_trailer1_axle1_roll  SampleTime=-1
  To Workspace3 : ToWorkspace  VariableName=p_trailer1_torsion  SampleTime=-1
  To Workspace30 : ToWorkspace  VariableName=p_trailer1_Fx  SampleTime=-1
  To Workspace31 : ToWorkspace  VariableName=p_trailer1_Fy  SampleTime=-1
  To Workspace4 : ToWorkspace  VariableName=p_trailer1_axle2_roll  SampleTime=-1
  To Workspace5 : ToWorkspace  VariableName=p_trailer1_axle1_pos  SampleTime=-1
  To Workspace6 : ToWorkspace  VariableName=p_trailer1_axle1_acc  SampleTime=-1
  To Workspace7 : ToWorkspace  VariableName=p_trailer1_omega  SampleTime=-1
  To Workspace8 : ToWorkspace  VariableName=p_trailer1_axle2_pos  SampleTime=-1
  To Workspace9 : ToWorkspace  VariableName=p_trailer1_Fz  SampleTime=-1
  wires:
  Bus Selector15/1 -> To Workspace17/1
  Bus Selector14/1 -> To Workspace16/1
  Bus Selector10/1 -> To Workspace23/1
  Bus Selector22/1 -> To Workspace1/1
  Bus Selector12/1 -> To Workspace10/1
  Bus Selector6/1 -> To Workspace6/1
  Bus Selector5/1 -> To Workspace5/1
  Subsystem3/1(Out1) -> To Workspace7/1
  Subsystem2/1(Out1) -> To Workspace9/1
  Subsystem1/1(Out1) -> To Workspace31/1
  Subsystem/1(Out1) -> To Workspace30/1
  Bus Selector3/1 -> To Workspace4/1
  Bus Selector2/1 -> To Workspace8/1
  Bus Selector11/1 -> To Workspace2/1
  Bus Selector7/1 -> To Workspace3/1
  Bus Selector1/1 -> To Workspace12/1
  In1/1 -> Bus Selector3/1, Bus Selector2/1, Bus Selector5/1, Bus Selector12/1, Bus Selector10/1, Bus Selector13/1, Bus Selector11/1, Bus Selector9/1, Bus Selector8/1, Bus Selector22/1, Bus Selector1/1, Bus Selector15/1, Bus Selector4/1, Subsystem2/1(In1), Subsystem3/1(In1), Bus Selector7/1, Subsystem1/1(In1), Subsystem/1(In1), Bus Selector14/1, Bus Selector6/1
  Bus Selector4/1 -> To Workspace11/1
  Bus Selector9/1 -> To Workspace14/1
  Bus Selector13/1 -> To Workspace15/1
  Bus Selector8/1 -> To Workspace13/1

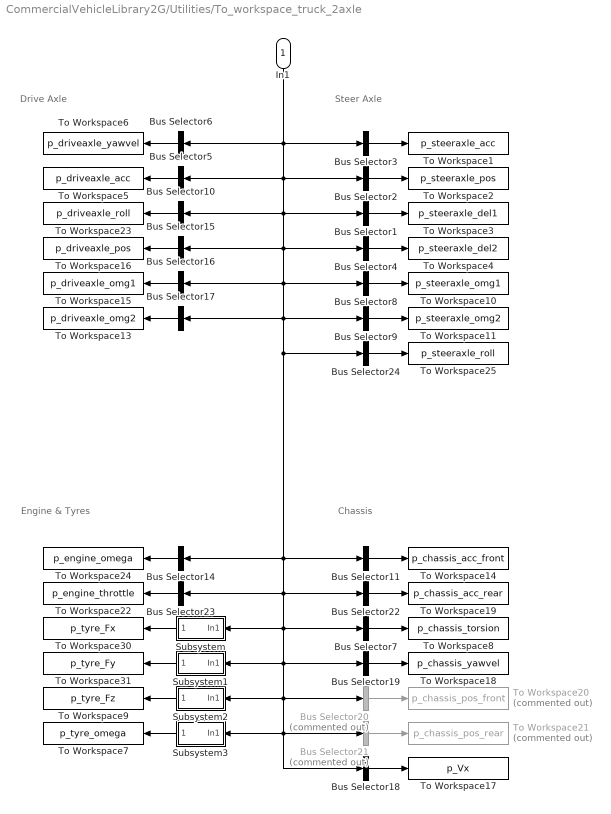
== system CommercialVehicleLibrary2G/Utilities/To_workspace_truck_2axle ==
  note: Engine & Tyres
  note: Chassis
  note: Steer Axle
  note: Drive Axle
  In1 : Inport
  Bus Selector1 : BusSelector  OutputSignals=steeraxle.Delta 1_L  OutputAsBus=on
  Bus Selector10 : BusSelector  OutputSignals=driveaxle.roll  OutputAsBus=on
  Bus Selector11 : BusSelector  OutputSignals=chassis.front_acc  OutputAsBus=on
  Bus Selector14 : BusSelector  OutputSignals=driveline.omega  OutputAsBus=on
  Bus Selector15 : BusSelector  OutputSignals=driveaxle.pos  OutputAsBus=on
  Bus Selector16 : BusSelector  OutputSignals=driveaxle.Omega1  OutputAsBus=on
  Bus Selector17 : BusSelector  OutputSignals=driveaxle.Omega2  OutputAsBus=on
  Bus Selector18 : BusSelector  OutputSignals=chassis.Vx  OutputAsBus=on
  Bus Selector19 : BusSelector  OutputSignals=chassis.yawvel  OutputAsBus=on
  Bus Selector2 : BusSelector  OutputSignals=steeraxle.pos  OutputAsBus=on
  Bus Selector20 : BusSelector  Commented=on  OutputSignals=chassis.G2_pos_chassis frt  OutputAsBus=on
  Bus Selector21 : BusSelector  Commented=on  OutputSignals=chassis.G2_pos_chassis rear  OutputAsBus=on
  Bus Selector22 : BusSelector  OutputSignals=chassis.centre_acc  OutputAsBus=on
  Bus Selector23 : BusSelector  OutputSignals=driveline.throttle  OutputAsBus=on
  Bus Selector24 : BusSelector  OutputSignals=steeraxle.roll  OutputAsBus=on
  Bus Selector3 : BusSelector  OutputSignals=steeraxle.acc  OutputAsBus=on
  Bus Selector4 : BusSelector  OutputSignals=steeraxle.Delta 2_R  OutputAsBus=on
  Bus Selector5 : BusSelector  OutputSignals=driveaxle.acc  OutputAsBus=on
  Bus Selector6 : BusSelector  OutputSignals=chassis.yawvel  OutputAsBus=on
  Bus Selector7 : BusSelector  OutputSignals=chassis.torsion  OutputAsBus=on
  Bus Selector8 : BusSelector  OutputSignals=steeraxle.Omega1  OutputAsBus=on
  Bus Selector9 : BusSelector  OutputSignals=steeraxle.Omega2  OutputAsBus=on
  Subsystem : Subsystem
  Subsystem1 : Subsystem
  Subsystem2 : Subsystem
  Subsystem3 : Subsystem
  To Workspace1 : ToWorkspace  VariableName=p_steeraxle_acc  SampleTime=-1
  To Workspace10 : ToWorkspace  VariableName=p_steeraxle_omg1  SampleTime=-1
  To Workspace11 : ToWorkspace  VariableName=p_steeraxle_omg2  SampleTime=-1
  To Workspace13 : ToWorkspace  VariableName=p_driveaxle_omg2  SampleTime=-1
  To Workspace14 : ToWorkspace  VariableName=p_chassis_acc_front  SampleTime=-1
  To Workspace15 : ToWorkspace  VariableName=p_driveaxle_omg1  SampleTime=-1
  To Workspace16 : ToWorkspace  VariableName=p_driveaxle_pos  SampleTime=-1
  To Workspace17 : ToWorkspace  VariableName=p_Vx  SampleTime=-1
  To Workspace18 : ToWorkspace  VariableName=p_chassis_yawvel  SampleTime=-1
  To Workspace19 : ToWorkspace  VariableName=p_chassis_acc_rear  SampleTime=-1
  To Workspace2 : ToWorkspace  VariableName=p_steeraxle_pos  SampleTime=-1
  To Workspace20 : ToWorkspace  Commented=on  VariableName=p_chassis_pos_front  SampleTime=-1
  To Workspace21 : ToWorkspace  Commented=on  VariableName=p_chassis_pos_rear  SampleTime=-1
  To Workspace22 : ToWorkspace  VariableName=p_engine_throttle  SampleTime=-1
  To Workspace23 : ToWorkspace  VariableName=p_driveaxle_roll  SampleTime=-1
  To Workspace24 : ToWorkspace  VariableName=p_engine_omega  SampleTime=-1
  To Workspace25 : ToWorkspace  VariableName=p_steeraxle_roll  SampleTime=-1
  To Workspace3 : ToWorkspace  VariableName=p_steeraxle_del1  SampleTime=-1
  To Workspace30 : ToWorkspace  VariableName=p_tyre_Fx  SampleTime=-1
  To Workspace31 : ToWorkspace  VariableName=p_tyre_Fy  SampleTime=-1
  To Workspace4 : ToWorkspace  VariableName=p_steeraxle_del2  SampleTime=-1
  To Workspace5 : ToWorkspace  VariableName=p_driveaxle_acc  SampleTime=-1
  To Workspace6 : ToWorkspace  VariableName=p_driveaxle_yawvel  SampleTime=-1
  To Workspace7 : ToWorkspace  VariableName=p_tyre_omega  SampleTime=-1
  To Workspace8 : ToWorkspace  VariableName=p_chassis_torsion  SampleTime=-1
  To Workspace9 : ToWorkspace  VariableName=p_tyre_Fz  SampleTime=-1
  wires:
  Bus Selector14/1 -> To Workspace24/1
  Bus Selector11/1 -> To Workspace14/1
  Bus Selector18/1 -> To Workspace17/1
  Bus Selector7/1 -> To Workspace8/1
  Bus Selector2/1 -> To Workspace2/1
  Bus Selector3/1 -> To Workspace1/1
  Subsystem/1(Out1) -> To Workspace30/1
  Subsystem1/1(Out1) -> To Workspace31/1
  Subsystem2/1(Out1) -> To Workspace9/1
  Subsystem3/1(Out1) -> To Workspace7/1
  Bus Selector1/1 -> To Workspace3/1
  Bus Selector4/1 -> To Workspace4/1
  Bus Selector5/1 -> To Workspace5/1
  Bus Selector6/1 -> To Workspace6/1
  Bus Selector8/1 -> To Workspace10/1
  Bus Selector9/1 -> To Workspace11/1
  Bus Selector16/1 -> To Workspace15/1
  Bus Selector17/1 -> To Workspace13/1
  Bus Selector15/1 -> To Workspace16/1
  Bus Selector19/1 -> To Workspace18/1
  Bus Selector22/1 -> To Workspace19/1
  In1/1 -> Bus Selector6/1, Bus Selector23/1, Bus Selector18/1, Subsystem3/1(In1), Bus Selector21/1, Subsystem2/1(In1), Bus Selector20/1, Subsystem1/1(In1), Bus Selector19/1, Subsystem/1(In1), Bus Selector7/1, Bus Selector22/1, Bus Selector14/1, Bus Selector11/1, Bus Selector24/1, Bus Selector17/1, Bus Selector9/1, Bus Selector16/1, Bus Selector8/1, Bus Selector15/1, Bus Selector4/1, Bus Selector1/1, Bus Selector10/1, Bus Selector5/1, Bus Selector2/1, Bus Selector3/1
  Bus Selector20/1 -> To Workspace20/1
  Bus Selector21/1 -> To Workspace21/1
  Bus Selector23/1 -> To Workspace22/1
  Bus Selector10/1 -> To Workspace23/1
  Bus Selector24/1 -> To Workspace25/1

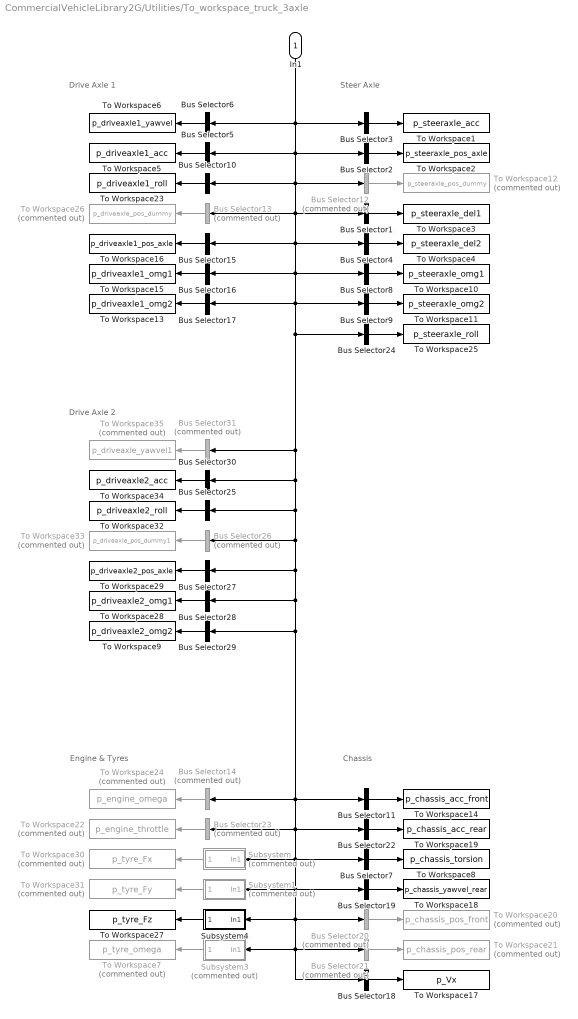
== system CommercialVehicleLibrary2G/Utilities/To_workspace_truck_3axle ==
  note: Engine & Tyres
  note: Chassis
  note: Steer Axle
  note: Drive Axle 1
  note: Drive Axle 2
  In1 : Inport
  Bus Selector1 : BusSelector  OutputSignals=steeraxle.Delta 1_L  OutputAsBus=on
  Bus Selector10 : BusSelector  OutputSignals=driveaxle1.roll  OutputAsBus=on
  Bus Selector11 : BusSelector  OutputSignals=chassis.front_acc  OutputAsBus=on
  Bus Selector12 : BusSelector  Commented=on  OutputSignals=steeraxle.Dummyaxle_pos  OutputAsBus=on
  Bus Selector13 : BusSelector  Commented=on  OutputSignals=driveaxle1.G2_Driveaxle_pos_dummy  OutputAsBus=on
  Bus Selector14 : BusSelector  Commented=on  OutputSignals=driveline.G2_omega_engine  OutputAsBus=on
  Bus Selector15 : BusSelector  OutputSignals=driveaxle1.pos  OutputAsBus=on
  Bus Selector16 : BusSelector  OutputSignals=driveaxle1.Omega1  OutputAsBus=on
  Bus Selector17 : BusSelector  OutputSignals=driveaxle1.Omega2  OutputAsBus=on
  Bus Selector18 : BusSelector  OutputSignals=chassis.Vx  OutputAsBus=on
  Bus Selector19 : BusSelector  OutputSignals=chassis.yawvel  OutputAsBus=on
  Bus Selector2 : BusSelector  OutputSignals=steeraxle.pos  OutputAsBus=on
  Bus Selector20 : BusSelector  Commented=on  OutputSignals=chassis.G2_pos_chassis frt  OutputAsBus=on
  Bus Selector21 : BusSelector  Commented=on  OutputSignals=chassis.G2_pos_chassis rear  OutputAsBus=on
  Bus Selector22 : BusSelector  OutputSignals=chassis.centre_acc  OutputAsBus=on
  Bus Selector23 : BusSelector  Commented=on  OutputSignals=driveline.G2_throttle_engine  OutputAsBus=on
  Bus Selector24 : BusSelector  OutputSignals=steeraxle.roll  OutputAsBus=on
  Bus Selector25 : BusSelector  OutputSignals=driveaxle2.roll  OutputAsBus=on
  Bus Selector26 : BusSelector  Commented=on  OutputSignals=driveaxle1.G2_Driveaxle_pos_dummy  OutputAsBus=on
  Bus Selector27 : BusSelector  OutputSignals=driveaxle2.pos  OutputAsBus=on
  Bus Selector28 : BusSelector  OutputSignals=driveaxle2.Omega1  OutputAsBus=on
  Bus Selector29 : BusSelector  OutputSignals=driveaxle2.Omega2  OutputAsBus=on
  Bus Selector3 : BusSelector  OutputSignals=steeraxle.acc  OutputAsBus=on
  Bus Selector30 : BusSelector  OutputSignals=driveaxle2.acc  OutputAsBus=on
  Bus Selector31 : BusSelector  Commented=on  OutputSignals=chassis.G2_yawvel_chassis_rear  OutputAsBus=on
  Bus Selector4 : BusSelector  OutputSignals=steeraxle.Delta 2_R  OutputAsBus=on
  Bus Selector5 : BusSelector  OutputSignals=driveaxle1.acc  OutputAsBus=on
  Bus Selector6 : BusSelector  OutputSignals=chassis.yawvel  OutputAsBus=on
  Bus Selector7 : BusSelector  OutputSignals=chassis.torsion  OutputAsBus=on
  Bus Selector8 : BusSelector  OutputSignals=steeraxle.Omega1  OutputAsBus=on
  Bus Selector9 : BusSelector  OutputSignals=steeraxle.Omega2  OutputAsBus=on
  Subsystem : Subsystem  Commented=on
  Subsystem1 : Subsystem  Commented=on
  Subsystem3 : Subsystem  Commented=on
  Subsystem4 : Subsystem
  To Workspace1 : ToWorkspace  VariableName=p_steeraxle_acc  SampleTime=-1
  To Workspace10 : ToWorkspace  VariableName=p_steeraxle_omg1  SampleTime=-1
  To Workspace11 : ToWorkspace  VariableName=p_steeraxle_omg2  SampleTime=-1
  To Workspace12 : ToWorkspace  Commented=on  VariableName=p_steeraxle_pos_dummy  SampleTime=-1
  To Workspace13 : ToWorkspace  VariableName=p_driveaxle1_omg2  SampleTime=-1
  To Workspace14 : ToWorkspace  VariableName=p_chassis_acc_front  SampleTime=-1
  To Workspace15 : ToWorkspace  VariableName=p_driveaxle1_omg1  SampleTime=-1
  To Workspace16 : ToWorkspace  VariableName=p_driveaxle1_pos_axle  SampleTime=-1
  To Workspace17 : ToWorkspace  VariableName=p_Vx  SampleTime=-1
  To Workspace18 : ToWorkspace  VariableName=p_chassis_yawvel_rear  SampleTime=-1
  To Workspace19 : ToWorkspace  VariableName=p_chassis_acc_rear  SampleTime=-1
  To Workspace2 : ToWorkspace  VariableName=p_steeraxle_pos_axle  SampleTime=-1
  To Workspace20 : ToWorkspace  Commented=on  VariableName=p_chassis_pos_front  SampleTime=-1
  To Workspace21 : ToWorkspace  Commented=on  VariableName=p_chassis_pos_rear  SampleTime=-1
  To Workspace22 : ToWorkspace  Commented=on  VariableName=p_engine_throttle  SampleTime=-1
  To Workspace23 : ToWorkspace  VariableName=p_driveaxle1_roll  SampleTime=-1
  To Workspace24 : ToWorkspace  Commented=on  VariableName=p_engine_omega  SampleTime=-1
  To Workspace25 : ToWorkspace  VariableName=p_steeraxle_roll  SampleTime=-1
  To Workspace26 : ToWorkspace  Commented=on  VariableName=p_driveaxle_pos_dummy  SampleTime=-1
  To Workspace27 : ToWorkspace  VariableName=p_tyre_Fz  SampleTime=-1
  To Workspace28 : ToWorkspace  VariableName=p_driveaxle2_omg1  SampleTime=-1
  To Workspace29 : ToWorkspace  VariableName=p_driveaxle2_pos_axle  SampleTime=-1
  To Workspace3 : ToWorkspace  VariableName=p_steeraxle_del1  SampleTime=-1
  To Workspace30 : ToWorkspace  Commented=on  VariableName=p_tyre_Fx  SampleTime=-1
  To Workspace31 : ToWorkspace  Commented=on  VariableName=p_tyre_Fy  SampleTime=-1
  To Workspace32 : ToWorkspace  VariableName=p_driveaxle2_roll  SampleTime=-1
  To Workspace33 : ToWorkspace  Commented=on  VariableName=p_driveaxle_pos_dummy1  SampleTime=-1
  To Workspace34 : ToWorkspace  VariableName=p_driveaxle2_acc  SampleTime=-1
  To Workspace35 : ToWorkspace  Commented=on  VariableName=p_driveaxle_yawvel1  SampleTime=-1
  To Workspace4 : ToWorkspace  VariableName=p_steeraxle_del2  SampleTime=-1
  To Workspace5 : ToWorkspace  VariableName=p_driveaxle1_acc  SampleTime=-1
  To Workspace6 : ToWorkspace  VariableName=p_driveaxle1_yawvel  SampleTime=-1
  To Workspace7 : ToWorkspace  Commented=on  VariableName=p_tyre_omega  SampleTime=-1
  To Workspace8 : ToWorkspace  VariableName=p_chassis_torsion  SampleTime=-1
  To Workspace9 : ToWorkspace  VariableName=p_driveaxle2_omg2  SampleTime=-1
  wires:
  Bus Selector14/1 -> To Workspace24/1
  Bus Selector11/1 -> To Workspace14/1
  Bus Selector18/1 -> To Workspace17/1
  Bus Selector7/1 -> To Workspace8/1
  Bus Selector2/1 -> To Workspace2/1
  Bus Selector3/1 -> To Workspace1/1
  Subsystem/1(Out1) -> To Workspace30/1
  Subsystem1/1(Out1) -> To Workspace31/1
  Subsystem3/1(Out1) -> To Workspace7/1
  Bus Selector1/1 -> To Workspace3/1
  Bus Selector4/1 -> To Workspace4/1
  Bus Selector5/1 -> To Workspace5/1
  Bus Selector6/1 -> To Workspace6/1
  Bus Selector8/1 -> To Workspace10/1
  Bus Selector9/1 -> To Workspace11/1
  Bus Selector12/1 -> To Workspace12/1
  Bus Selector16/1 -> To Workspace15/1
  Bus Selector17/1 -> To Workspace13/1
  Bus Selector15/1 -> To Workspace16/1
  Bus Selector19/1 -> To Workspace18/1
  Bus Selector22/1 -> To Workspace19/1
  Bus Selector20/1 -> To Workspace20/1
  Bus Selector21/1 -> To Workspace21/1
  Bus Selector23/1 -> To Workspace22/1
  Bus Selector10/1 -> To Workspace23/1
  Bus Selector24/1 -> To Workspace25/1
  Bus Selector13/1 -> To Workspace26/1
  Subsystem4/1(Out1) -> To Workspace27/1
  Bus Selector26/1 -> To Workspace33/1
  Bus Selector25/1 -> To Workspace32/1
  In1/1 -> Bus Selector6/1, Bus Selector24/1, Bus Selector31/1, Bus Selector30/1, Bus Selector25/1, Bus Selector26/1, Bus Selector27/1, Bus Selector28/1, Bus Selector29/1, Bus Selector23/1, Subsystem4/1(In1), Bus Selector18/1, Subsystem3/1(In1), Bus Selector21/1, Bus Selector20/1, Subsystem1/1(In1), Bus Selector19/1, Subsystem/1(In1), Bus Selector7/1, Bus Selector22/1, Bus Selector14/1, Bus Selector11/1, Bus Selector17/1, Bus Selector9/1, Bus Selector16/1, Bus Selector8/1, Bus Selector15/1, Bus Selector4/1, Bus Selector13/1, Bus Selector1/1, Bus Selector10/1, Bus Selector12/1, Bus Selector5/1, Bus Selector2/1, Bus Selector3/1
  Bus Selector27/1 -> To Workspace29/1
  Bus Selector29/1 -> To Workspace9/1
  Bus Selector28/1 -> To Workspace28/1
  Bus Selector31/1 -> To Workspace35/1
  Bus Selector30/1 -> To Workspace34/1
